simulink model "MCU_regionalPolePlacementLMI_SAME54_MCLV2"  (R2023b)
settings: Solver=FixedStepDiscrete  StartTime=0.0  StopTime=10.0  FixedStep=5e-5  RelTol=1e-3  EnableMultiTasking=on
InitFcn:
  | % DC Voltage
  | VDC = 24;
  | 
  | % Intersective PMW
  | Vmax = VDC/2;
  | Imax = 4;
  | 
  | Ts = 1e-4;
  | 
  | % pole paires
  | p = 4;
  | 
  | % QEI
  | lines = 4*1000;
  | eleclines = lines/p;
  | inveleclines = 1/eleclines
  | gainQEIspeed = 2*pi/Ts/lines
  | 
  | model.R = 0.656;         % Ohm
  | model.L = 0.35e-3;       % H
  | model.Phif = 6.6e-3;     % Wb
  | model.p = 4;
  | model.F = 1.e-05;
  | model.J = 1e-05;
  | disp(model);
  | 
  | % State space representation of the motor model
  | 
  | A = [-model.R/model.L -model.p*model.Phif ; 3*model.p*model.Phif/(2*model.J) -model.F/model.J ];
  | B = [1/model.L;0];
  | C = [0 1];
  | n=size(A,1);
  | % Augmented model with integral action
  | 
  | n=size(A,1); mx=size(B,2);
  | 
  | warning('off')
  | A = [A zeros(n,1);-C 0] ;
  | Bu=[B;0];Bw=[eye(3)];Duz=[1];Cz=[0 0 0];
  | 
  | n= 3;
  | m = 1;
  | 
  | %%% LIST OF UKNOWNS (lambda is the first, always included)
  | Nunk=uint16(2);
  | nunk = 1;
  | %UNK=cell(Nunk,1);
  | UNK = struct(...
  |     ...%'lab',{'X','Y'},...
  |     'col',{uint16(n),uint16(n)},...
  |     'row',{uint16(n),uint16(m)},...
  |     'sym',{uint16(1),uint16(0)},...
  |     'start',{uint16(0),uint16(0)},...
  |     'siz',{uint16(n*(n+1)/2),uint16(n*m)},...
  |     'X',{single(zeros(n,n,n*(n+1)/2)),single(zeros(m,n,n*m))},...
  |     'ste',{single(zeros(n,n)),single(zeros(m,n))},...
  |     'end',{uint16(nunk),uint16(nunk)}...
  |    );
  | 
  | 
  | ... (+100 lines)
undefined symbols (not defined in the file or in its folder): ADC0, AIN0, AIN6, B27, DiscIntNeverNeededParam, NumBits1, NumBits2, PA02, PA03, PA06, PA08, PA09, PA10, PA11, PA12, PA13, PA16, PA17, PA18, pad0, pad1, pad2, pad3, PB08, PC16, PC17, PC18, Pin, SAME54P20A, TQFP128, VREFA, wo0, wo1, wo2, wo4, wo5, wo6
libraries: simulink x20, MCHP_Blockset x12, dspfdesign x1
(part 3 of 3)

== matlab function MCU_regionalPolePlacementLMI_SAME54_MCLV2/Gains Tunning/Subsystem5/Subsystem/MATLAB Function2 ==
  settings: updateMethod=DISCRETE
  data: A input single; B input single; alpha input single; K1 output single; K2 output single; K3 output single; UNK input; F input; FINV input; FF input; FFF input; V input
function [K1,K2,K3]=fcn(A,B,alpha,UNK,F,FINV,FF,FFF,V)
K1 = single(0);
K2 = single(0);
K3 = single(0);
U ={"UNK1","UNK2"};
FFname ={"Ft1","Ft2","Ft3","Ft4"};
FFFname ={"Ft1x","Ft2x","Ft3x","Ft4x"};

Ncon=uint16(4);
maxeig=single(zeros(Ncon+1,1));
%alpha = single(20);
beta=single(1);
tol = single(1e-3);
Bu=single([B;0]);Bw=single([eye(3)]);Duz=single([1]);Cz=single([0 0 0]);
X = single(zeros(3));
Y = single(zeros(1,3));

Nunk = single(2);
nunk = single(10);

alphamax = 3*alpha;
grad=single(zeros(nunk,1));
hess=single(zeros(nunk,nunk));

it=single(0);
jj=single(0);


for i=1:nunk+1

    for j=1:Nunk
        UNK.(U{j}).ste=0*UNK.(U{j}).ste;
    end

    for j=1:Nunk


        if i >= UNK.(U{j}).start && i <= UNK.(U{j}).end
            break
        end
    end
    if j>Nunk && i~=nunk+1

        error('');

    end
    for l=1:2

        if l==2 && i~=nunk+1 && i~=1
            %disp('in')
            for k=1:Nunk
                if(k == j)
                    %disp(i-single(UNK.(U{k}).start))
                    UNK.(U{k}).ste=UNK.(U{k}).X(:,:,i-single(UNK.(U{k}).start)+1);
                end
            end
        end



        X=UNK.UNK1.ste
        Y=UNK.UNK2.ste
        FF.Ft1(l).X= X;
        FF.Ft2(l).X= [-B*Y-Y'*B'-2*alpha*X-X*A'-A*X];
        FF.Ft3(l).X= B*Y+Y'*B'+2*alphamax*X+X*A'+A*X;
        FF.Ft4(l).X= -[beta*(X*A'+A*X)  A*X-X*A'; (A*X-X*A')'  beta*(X*A'+A*X)]-...
                    [beta*(Y'*B'+B*Y)  B*Y-Y'*B'; ( B*Y-Y'*B')'  beta*(Y'*B'+B*Y)]; 
        %FF.Ft8(1,l).X
    end

    for c=1:Ncon

        if i==nunk+1 %%% F0 constant term
            FFF.(FFFname{c})(i).X = FF.(FFname{c})(1).X;
            %F(c,i).X=Ft(c,1).X;
            maxeig(c)=single(min(real(eig(FFF.(FFFname{c})(i).X))));
        elseif i==1
            if c==Ncon+1
                FFF.(FFFname{c})(i).X=single(-1); %%% lambda term on additional constraint (lambda < 0) for opt
            else
                FFF.(FFFname{c})(i).X=single(eye(size(FF.(FFname{c})(2).X,2)));  %%% lambda term for feas
            end
        else
            FFF.(FFFname{c})(i).X = FF.(FFname{c})(2).X-FF.(FFname{c})(1).X;

            %F(c,i).X=Ft(c,2).X-Ft(c,1).X;       %%% standard terms
        end
    end

end

%%
%x= single([-min([min(maxeig) 0])+0.1; zeros(nunk-2,1); 100]); % [-min([min(maxeig) 0])+1; zeros(nunk-2,1); 1000]; %initial conditions
theta=0;%.1;
x0=[-min([min(maxeig) 0])+1; zeros(nunk-1,1)];


it=0;
x=x0;
t=1;

disp('start optim');
while 1
    it=it+1;
    disp(it);
    x00=x;
    j=0;
    while 1
        x0=x;
        j=j+1;
        %disp(j);
        grad=0*x;


        for c=1:Ncon
            FF.(FFname{c})(1).X = FFF.(FFFname{c})(11).X;
            %disp(FFF.(FFFname{c})(18).X)
            %pause

            for i=1:nunk
               
                FF.(FFname{c})(1).X = FF.(FFname{c})(1).X + x(i)*FFF.(FFFname{c})(i).X;
                %                Ft(c,1).X=Ft(c,1).X+x(i)*F(c,i).X;
            end

            F.(FFname{c}).X=FF.(FFname{c})(1).X;
            FINV.(FFname{c}).X=F.(FFname{c}).X^-1;
            %disp(FINV.(FFname{c}).X)
            %pause
        end


        for i=1:nunk
            for c=1:Ncon
                V.(FFFname{c})(i).X=FINV.(FFname{c}).X*FFF.(FFFname{c})(i).X;
                grad(i)=grad(i)-trace(V.(FFFname{c})(i).X);
            end
        end

            grad(1)=grad(1)+t ;
        
        hess=hess*0;
        for i=1:nunk
            for ii=i:nunk
                for c=1:Ncon
                    hess(i,ii)=hess(i,ii)+trace(V.(FFFname{c})(i).X*V.(FFFname{c})(ii).X);
                    if i~=ii && c==Ncon
                        hess(ii,i)=hess(i,ii);
                    end
                end
            end
        end

        
        % if flag
        %keyboard

        %x=x - single(double(hess)\double(grad)*0.1);  %x=x- pinv(hess)*grad;
        x=x - ((hess)\(grad));  %x=x- pinv(hess)*grad;
        %      [x(1) x(end)]
        %     if (isnan(x(1)))
        %     error("NaN algo diverge ")
        %     end
        %     %keyboard;
        %else
        %     x(2:end)=x(2:end)- hess(2:end,2:end)\grad(2:end);
        % end
        %

        if norm(x-x00)<=tol || x(1)<=-tol%1
            break;
       end
       x00=x;     
   end 

   
   if norm(x-x0)<=tol || x(1)<=-tol %1
       break;
   end
   %l0=theta*(x0(1))+(1-theta)*l;
   t=1.5*t;
   x0=x;


end


    %if  x(1)<= 0
    %disp('feasible problem');
    for j=1:Nunk
        UNK.(U{j}).ste=0*UNK.(U{j}).ste;
    end



    for i=2:nunk

        for j=1:Nunk
            if i >= UNK.(U{j}).start && i <= UNK.(U{j}).end
                UNK.(U{j}).ste=UNK.(U{j}).ste+x(i)*UNK.(U{j}).X(:,:,i-single(UNK.(U{j}).start)+1);
                break
            end
        end

    end

    %else
    %    disp('infeasible problem');
    %end

    X=UNK.(U{1}).ste;
    Y=UNK.(U{2}).ste;
    P=X^-1;
    K=Y*P;
    K1 = K(1);
    K2 = K(2);
    K3 = K(3);
